simulink model "CLLLC_backward"  (R2018a)
settings: Solver=ode23tb  StartTime=0.0  StopTime=0.2  RelTol=1e-3
undefined symbols (not defined in the file): Lm
libraries: powerlib x49
settings Model: Creator=sy167  LastModifiedBy=sy167

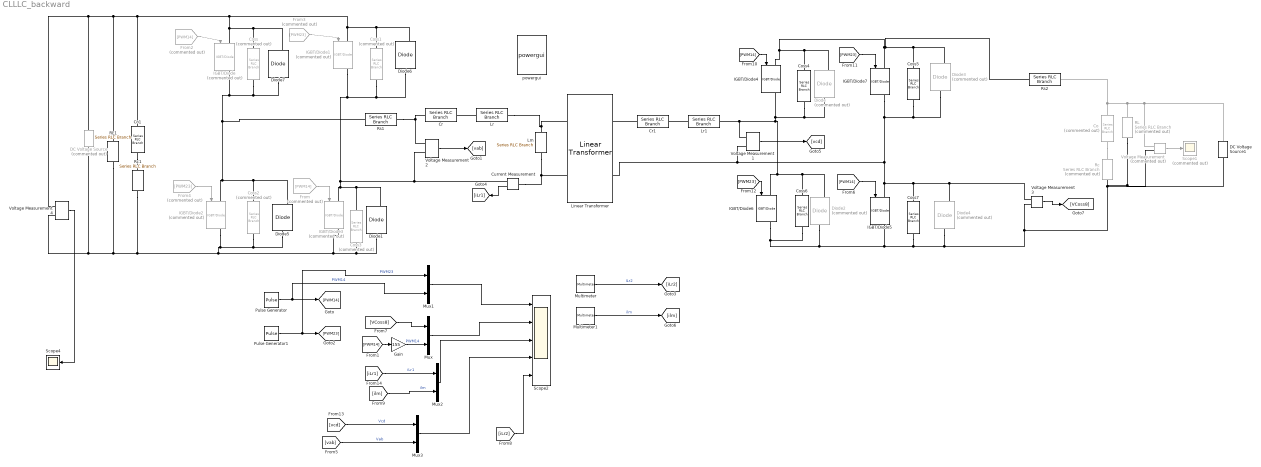
== system CLLLC_backward ==
  Co : powerlib/Elements/Series RLC Branch  Commented=on  LConnTagsString=__new0  RConnTagsString=__new0  BranchType=C  Resistance=1  Inductance=72e-6  SetiL0=off  InitialCurrent=0  Capacitance=2200e-6  Setx0=off  InitialVoltage=1500  Measurements=Branch voltage
  Co1 : powerlib/Elements/Series RLC Branch  LConnTagsString=__new0  RConnTagsString=__new0  BranchType=C  Resistance=1  Inductance=72e-6  SetiL0=off  InitialCurrent=0  Capacitance=2200e-6  Setx0=off  InitialVoltage=1500  Measurements=Branch voltage
  Coss : powerlib/Elements/Series RLC Branch  Commented=on  LConnTagsString=__new0  RConnTagsString=__new0  BranchType=C  Resistance=1  Inductance=72e-6  SetiL0=off  InitialCurrent=0  Capacitance=1000e-12  Setx0=off  InitialVoltage=0  Measurements=None
  Coss1 : powerlib/Elements/Series RLC Branch  Commented=on  LConnTagsString=__new0  RConnTagsString=__new0  BranchType=C  Resistance=1  Inductance=72e-6  SetiL0=off  InitialCurrent=0  Capacitance=1000e-12  Setx0=off  InitialVoltage=0  Measurements=None
  Coss2 : powerlib/Elements/Series RLC Branch  Commented=on  LConnTagsString=__new0  RConnTagsString=__new0  BranchType=C  Resistance=1  Inductance=72e-6  SetiL0=off  InitialCurrent=0  Capacitance=1000e-12  Setx0=off  InitialVoltage=0  Measurements=None
  Coss3 : powerlib/Elements/Series RLC Branch  Commented=on  LConnTagsString=__new0  RConnTagsString=__new0  BranchType=C  Resistance=1  Inductance=72e-6  SetiL0=off  InitialCurrent=0  Capacitance=1000e-12  Setx0=off  InitialVoltage=0  Measurements=Branch current
  Coss4 : powerlib/Elements/Series RLC Branch  LConnTagsString=__new0  RConnTagsString=__new0  BranchType=C  Resistance=1  Inductance=72e-6  SetiL0=off  InitialCurrent=0  Capacitance=1000e-12  Setx0=off  InitialVoltage=0  Measurements=None
  Coss5 : powerlib/Elements/Series RLC Branch  LConnTagsString=__new0  RConnTagsString=__new0  BranchType=C  Resistance=1  Inductance=72e-6  SetiL0=off  InitialCurrent=0  Capacitance=1000e-12  Setx0=off  InitialVoltage=0  Measurements=None
  Coss6 : powerlib/Elements/Series RLC Branch  LConnTagsString=__new0  RConnTagsString=__new0  BranchType=C  Resistance=1  Inductance=72e-6  SetiL0=off  InitialCurrent=0  Capacitance=1000e-12  Setx0=off  InitialVoltage=0  Measurements=None
  Coss7 : powerlib/Elements/Series RLC Branch  LConnTagsString=__new0  RConnTagsString=__new0  BranchType=C  Resistance=1  Inductance=72e-6  SetiL0=off  InitialCurrent=0  Capacitance=1000e-12  Setx0=off  InitialVoltage=0  Measurements=Branch current
  Cr : powerlib/Elements/Series RLC Branch  LConnTagsString=__new0  RConnTagsString=__new0  BranchType=C  Resistance=1  Inductance=72e-6  SetiL0=off  InitialCurrent=0  Capacitance=31.4e-9  Setx0=off  InitialVoltage=0  Measurements=None
  Cr1 : powerlib/Elements/Series RLC Branch  LConnTagsString=__new0  RConnTagsString=__new0  BranchType=C  Resistance=1  Inductance=72e-6  SetiL0=off  InitialCurrent=0  Capacitance=1.3e-6  Setx0=off  InitialVoltage=0  Measurements=Branch current
  Current Measurement : powerlib/Measurements/Current Measurement  PhasorSimulation=off  OutputType=Complex  PSBequivalent=0
  DC Voltage Source : powerlib/Electrical Sources/DC Voltage Source  Commented=on  Amplitude=311  Measurements=None
  DC Voltage Source1 : powerlib/Electrical Sources/DC Voltage Source  Amplitude=48  Measurements=None
  Diode{,2..4} (4 alike) : powerlib/Power Electronics/Diode  Commented=on  Ron=0.001  Lon=0  Vf=0.8  IC=0  UseSnubber=0  Rs=500  Cs=250e-9  Measurements=on
  Diode{1,5..7} (4 alike) : powerlib/Power Electronics/Diode  Ron=0.001  Lon=0  Vf=0.8  IC=0  UseSnubber=0  Rs=500  Cs=250e-9  Measurements=on
  From : From  Commented=on  GotoTag=PWM14
  From2 : From  Commented=on  GotoTag=PWM14
  From3 : From  Commented=on  GotoTag=PWM23
  From4 : From  Commented=on  GotoTag=PWM23
  Gain : Gain  Gain=155
  IGBT/Diode{,1..3} (4 alike) : powerlib/Power Electronics/IGBT//Diode  Commented=on  Ron=1e-3  Rs=1e5  Cs=inf  Measurements=on
  IGBT/Diode{4..7} (4 alike) : powerlib/Power Electronics/IGBT//Diode  Ron=1e-3  Rs=1e5  Cs=inf  Measurements=on
  Linear Transformer : powerlib/Elements/Linear Transformer  UNITS=SI  NominalPower=[ 250e6 100e3]  winding1=[6.5 0 0]  winding2=[1 0 0]  ThreeWindings=off  winding3=[1 0 0]  RmLm=[1e6 inf]  Measurements=None  DataType=on
  Lm : powerlib/Elements/Series RLC Branch  LConnTagsString=__new0  RConnTagsString=__new0  BranchType=L  Resistance=1  Inductance=201.725e-6  SetiL0=off  InitialCurrent=0  Capacitance=1e-6  Setx0=off  InitialVoltage=0  Measurements=Branch current
  Lr : powerlib/Elements/Series RLC Branch  LConnTagsString=__new0  RConnTagsString=__new0  BranchType=L  Resistance=1  Inductance=80.7e-6  SetiL0=off  InitialCurrent=0  Capacitance=1e-6  Setx0=off  InitialVoltage=0  Measurements=None
  Lr1 : powerlib/Elements/Series RLC Branch  LConnTagsString=__new0  RConnTagsString=__new0  BranchType=L  Resistance=1  Inductance=1.9e-6  SetiL0=off  InitialCurrent=0  Capacitance=1e-6  Setx0=off  InitialVoltage=0  Measurements=Branch current
  Multimeter : powerlib/Measurements/Multimeter  PhasorSimulation=off  OutputType=Complex  sel=5  L=7  Gain=1  yselected={'Ib: Lr1'};  PSBOutputType=1  PSBequivalent=0  AxesSetting=[0,0.1,-100,100]  Display=0  SavedBlockNames=-11
  Multimeter1 : powerlib/Measurements/Multimeter  PhasorSimulation=off  OutputType=Complex  sel=4  L=7  Gain=1  yselected={'Ib: Lm'};  PSBOutputType=1  PSBequivalent=0  AxesSetting=[0,0.1,-100,100]  Display=0  SavedBlockNames=-11
  Mux{,1..3} (4 alike) : Mux  Inputs=2
  Pulse Generator : DiscretePulseGenerator  PulseType=Time based  Period=1/110e3  PulseWidth=45
  Pulse Generator1 : DiscretePulseGenerator  PulseType=Time based  Period=1/110e3  PulseWidth=45  PhaseDelay=1/110e3/2
  RL : powerlib/Elements/Series RLC Branch  Commented=on  LConnTagsString=__new0  RConnTagsString=__new0  BranchType=R  Resistance=(48*48)/1000  Inductance=Lm  SetiL0=off  InitialCurrent=0  Capacitance=1e-6  Setx0=off  InitialVoltage=0  Measurements=None
  RL1 : powerlib/Elements/Series RLC Branch  LConnTagsString=__new0  RConnTagsString=__new0  BranchType=R  Resistance=97  Inductance=Lm  SetiL0=off  InitialCurrent=0  Capacitance=1e-6  Setx0=off  InitialVoltage=0  Measurements=None
  Rc : powerlib/Elements/Series RLC Branch  Commented=on  LConnTagsString=__new0  RConnTagsString=__new0  BranchType=R  Resistance=5e-3  Inductance=Lm  SetiL0=off  InitialCurrent=0  Capacitance=1e-6  Setx0=off  InitialVoltage=0  Measurements=None
  Rc1 : powerlib/Elements/Series RLC Branch  LConnTagsString=__new0  RConnTagsString=__new0  BranchType=R  Resistance=5e-3  Inductance=Lm  SetiL0=off  InitialCurrent=0  Capacitance=1e-6  Setx0=off  InitialVoltage=0  Measurements=None
  Rs1 : powerlib/Elements/Series RLC Branch  LConnTagsString=__new0  RConnTagsString=__new0  BranchType=R  Resistance=1e-6  Inductance=6.45e-6  SetiL0=off  InitialCurrent=0  Capacitance=1e-6  Setx0=off  InitialVoltage=0  Measurements=Branch current
  Rs2 : powerlib/Elements/Series RLC Branch  LConnTagsString=__new0  RConnTagsString=__new0  BranchType=R  Resistance=1e-6  Inductance=6.45e-6  SetiL0=off  InitialCurrent=0  Capacitance=1e-6  Setx0=off  InitialVoltage=0  Measurements=Branch current
  Scope1 : Scope  Commented=on
  Scope2 : Scope  NumInputPorts=5
  Scope4 : Scope
  Voltage Measurement : powerlib/Measurements/Voltage Measurement  Commented=on  PhasorSimulation=off  OutputType=Complex  PSBequivalent=0
  Voltage Measurement{1..4} (4 alike) : powerlib/Measurements/Voltage Measurement  PhasorSimulation=off  OutputType=Complex  PSBequivalent=0
  powergui : powerlib/powergui  Priority=1  SimulationMode=Discrete  SampleTime=1/200e3/1000  frequency=60  Iterations=50  frequencyindice=0  Pbase=100e6  ErrMax=1e-4  UnitsV=kV  UnitsW=MW  buscounter=0  FunctionMessages=off  echomessages=off  EnableUseOfTLC=off  CurrentSourceSwitches=off  DisableSnubberDevices=off  DisableRonSwitches=off  DisableVfSwitches=off  DisplayEquations=off  SolverType=Tustin/Backward Euler (TBE)  Interpol=off  ExternalGateDelay=off  methode=off  Ts=100  x0status=blocks  SPID=off  SwTol=0  HookPort=off  RestoreLinks=warning  ResistiveCurrentMeasurement=off  Frange=[0:2:500]  Ylog=off  Xlog=on  ShowGrid=off  save=off  variable=ZData  structure=0  ZoomFFT=on  StartTime=0.0  cycles=1  DisplayStyle=1  fundamental=60  FreqAxis=off  MaxFrequency=1000  frequencyindicesteady=1  RmsSteady=1  display=off
  wires:
  Multimeter1/1 -> [ilm]  "ilm"
  [iLr1] -> Mux2/1  "iLr1"
  Mux2/1 -> Scope2/3
  Current Measurement/1 -> [iLr1]
  [PWM14] -> IGBT/Diode4/1
  Multimeter/1 -> [iLr2]  "ILr2"
  [ilm] -> Mux2/2  "ilm"
  Voltage Measurement2/1 -> [vab]
  Pulse Generator/1 -> Mux1/2, [PWM14]  "PWM14"
  [PWM23] -> IGBT/Diode6/1
  From4/1 -> IGBT/Diode2/1
  From3/1 -> IGBT/Diode1/1
  Voltage Measurement/1 -> Scope1/1
  Gain/1 -> Mux/2  "PWM14"
  From/1 -> IGBT/Diode3/1
  [PWM14] -> Gain/1
  From2/1 -> IGBT/Diode/1
  Pulse Generator1/1 -> [PWM23], Mux1/1  "PWM23"
  [PWM14] -> IGBT/Diode5/1
  Mux/1 -> Scope2/2
  [PWM23] -> IGBT/Diode7/1
  Voltage Measurement3/1 -> [VCoss8]
  Voltage Measurement4/1 -> Scope4/1
  [VCoss8] -> Mux/1
  Voltage Measurement1/1 -> [vcd]
  Mux3/1 -> Scope2/4
  [vcd] -> Mux3/1  "Vcd"
  Mux1/1 -> Scope2/1
  [vab] -> Mux3/2  "Vab"
  [iLr2] -> Scope2/5
  connections:
  DC Voltage Source1/LConn1 -- IGBT/Diode5/RConn1 -- Diode2/LConn1 -- IGBT/Diode6/RConn1 -- Coss6/RConn1 -- Coss7/RConn1 -- Diode4/LConn1 -- Voltage Measurement3/LConn2 -- Rc/RConn1 -- RL/RConn1 -- Voltage Measurement/LConn2
  Coss5/LConn1 -- Diode3/RConn1 -- Rs2/LConn1 -- IGBT/Diode4/LConn1 -- Diode/RConn1 -- Coss4/LConn1 -- IGBT/Diode7/LConn1
  IGBT/Diode7/RConn1 -- Diode3/LConn1 -- Coss5/RConn1 -- Voltage Measurement1/LConn2 -- Linear Transformer/RConn2 -- Coss7/LConn1 -- Diode4/RConn1 -- Voltage Measurement3/LConn1 -- IGBT/Diode5/LConn1
  Rc1/RConn1 -- RL1/RConn1 -- Voltage Measurement4/LConn2 -- DC Voltage Source/LConn1 -- Diode5/LConn1 -- Coss2/RConn1 -- IGBT/Diode2/RConn1 -- Diode1/LConn1 -- Coss3/RConn1 -- IGBT/Diode3/RConn1
  Voltage Measurement2/LConn1 -- Cr/LConn1 -- Rs1/RConn1
  Current Measurement/RConn1 -- Voltage Measurement2/LConn2 -- Diode6/LConn1 -- Coss1/RConn1 -- IGBT/Diode1/RConn1 -- Coss3/LConn1 -- Diode1/RConn1 -- IGBT/Diode3/LConn1
  RL1/LConn1 -- Voltage Measurement4/LConn1 -- DC Voltage Source/RConn1 -- Diode6/RConn1 -- Coss1/LConn1 -- IGBT/Diode1/LConn1 -- IGBT/Diode/LConn1 -- Coss/LConn1 -- Diode7/RConn1 -- Co1/LConn1
  Current Measurement/LConn1 -- Linear Transformer/LConn2 -- Lm/RConn1
  Lr/RConn1 -- Linear Transformer/LConn1 -- Lm/LConn1
  Co/RConn1 -- Rc/LConn1
  Lr1/LConn1 -- Cr1/RConn1
  Cr1/LConn1 -- Linear Transformer/RConn1
  Lr/LConn1 -- Cr/RConn1
  Co1/RConn1 -- Rc1/LConn1
  IGBT/Diode6/LConn1 -- Voltage Measurement1/LConn1 -- Lr1/RConn1 -- Diode/LConn1 -- Coss4/RConn1 -- IGBT/Diode4/RConn1 -- Diode2/RConn1 -- Coss6/LConn1
  Voltage Measurement/LConn1 -- DC Voltage Source1/RConn1 -- Rs2/RConn1 -- Co/LConn1 -- RL/LConn1
  Diode7/LConn1 -- Coss/RConn1 -- IGBT/Diode/RConn1 -- Rs1/LConn1 -- IGBT/Diode2/LConn1 -- Coss2/LConn1 -- Diode5/RConn1
